simulink model "robotarm_core"  (R2025b)
settings: Solver=ode45  StartTime=0.0  StopTime=15  RelTol=1e-3
values from neighbouring files (symbols this model uses):
  d = 0.1    [params.m]
  g = 9.81    [params.m]
  l = 0.5    [params.m]
  m = 1.0    (= 1)    [params.m]
settings Model: Creator=alper  LastModifiedBy=alper
settings DebuggingCC: AlgebraicLoopMsg=none

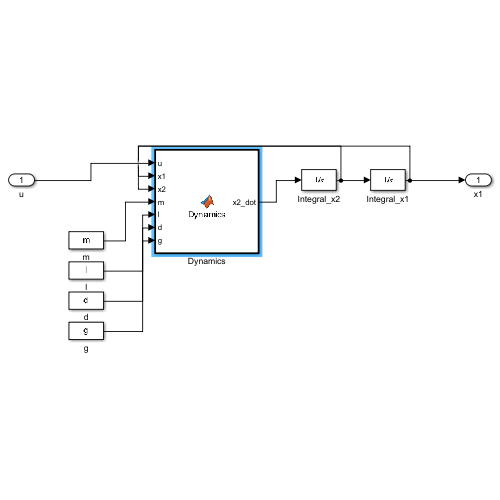
[thumbnail: Simulink's stored preview of the top-level diagram]
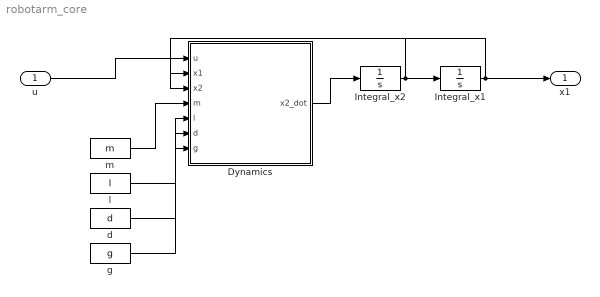
== system robotarm_core ==
  u : Inport
  Dynamics : MATLAB Function  TreatAsAtomicUnit=on
  Integral_x1 : Integrator
  Integral_x2 : Integrator
  d : Constant  Value=d
  g : Constant  Value=g
  l : Constant  Value=l
  m : Constant  Value=m
  x1 : Outport
  wires:
  u/1 -> Dynamics/1(u)
  m/1 -> Dynamics/4(m)
  l/1 -> Dynamics/5(l)
  d/1 -> Dynamics/6(d)
  g/1 -> Dynamics/7(g)
  Dynamics/1(x2_dot) -> Integral_x2/1
  Integral_x2/1 -> Integral_x1/1, Dynamics/3(x2)
  Integral_x1/1 -> Dynamics/2(x1), x1/1

== matlab function robotarm_core/Dynamics ==
  data: u input; x2_dot output; x1 input; x2 input; m input; l input; d input; g input
function x2_dot = Dynamics(u, x1, x2, m, l, d, g)
    x2_dot = robot_dynamics(u, x1, x2, m, l, d, g);
end
